simulink model "closed_loop_pd"  (R2023b)
settings: Solver=VariableStepAuto  StartTime=0.0  StopTime=0.15  RelTol=1e-3
undefined symbols (not defined in the file): a_m, config, K, K_g, K_m, K_pot, Kpd
settings Model: Creator=foderking  LastModifiedBy=foderking

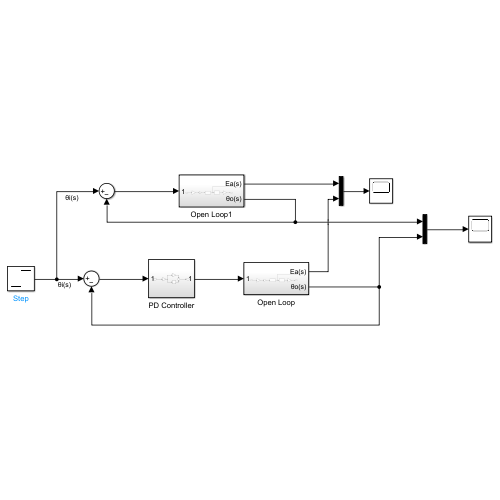
[thumbnail: Simulink's stored preview of the top-level diagram]
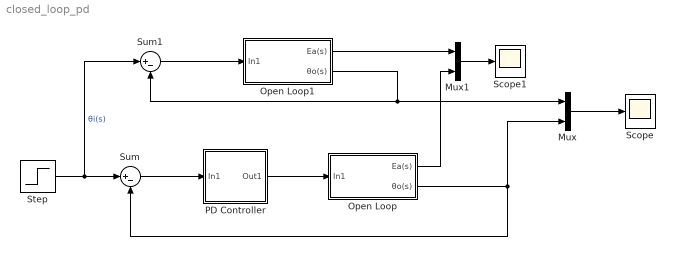
== system closed_loop_pd ==
  Mux : Mux  Inputs=2
  Mux1 : Mux  Inputs=2
  Open Loop : Subsystem
  Open Loop1 : Subsystem
  PD Controller : Subsystem
  Scope : Scope
  Scope1 : Scope
  Step : Step  Time=0  SampleTime=0
  Sum : Sum  Inputs=|+-
  Sum1 : Sum  Inputs=|+-
  wires:
  Open Loop/2(θo(s)) -> Sum/2, Mux/2
  Open Loop/1(Ea(s)) -> Mux1/2
  Step/1 -> Sum1/1, Sum/1  "θi(s)"
  Sum1/1 -> Open Loop1/1(In1)
  Open Loop1/1(Ea(s)) -> Mux1/1
  Open Loop1/2(θo(s)) -> Mux/1, Sum1/2
  Mux/1 -> Scope/1
  Sum/1 -> PD Controller/1(In1)
  PD Controller/1(Out1) -> Open Loop/1(In1)
  Mux1/1 -> Scope1/1

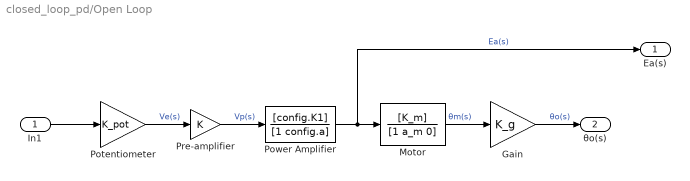
== system closed_loop_pd/Open Loop ==
  In1 : Inport
  Gain : Gain  Gain=K_g
  Motor : TransferFcn  Numerator=[K_m]  Denominator=[1 a_m 0]
  Potentiometer : Gain  Gain=K_pot
  Power Amplifier : TransferFcn  Numerator=[config.K1]  Denominator=[1 config.a]
  Pre-amplifier : Gain  Gain=K
  Ea(s) : Outport
  θo(s) : Outport  Port=2
  wires:
  Power Amplifier/1 -> Ea(s)/1, Motor/1  "Ea(s)"
  Potentiometer/1 -> Pre-amplifier/1  "Ve(s)"
  Motor/1 -> Gain/1  "θm(s)"
  In1/1 -> Potentiometer/1
  Pre-amplifier/1 -> Power Amplifier/1  "Vp(s)"
  Gain/1 -> θo(s)/1  "θo(s)"

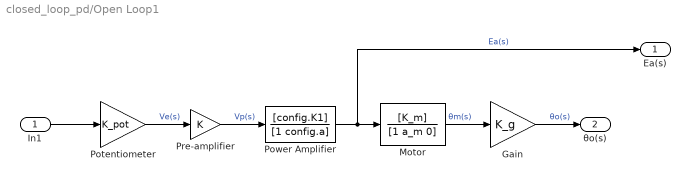
== system closed_loop_pd/Open Loop1 ==
  In1 : Inport
  Gain : Gain  Gain=K_g
  Motor : TransferFcn  Numerator=[K_m]  Denominator=[1 a_m 0]
  Potentiometer : Gain  Gain=K_pot
  Power Amplifier : TransferFcn  Numerator=[config.K1]  Denominator=[1 config.a]
  Pre-amplifier : Gain  Gain=K
  Ea(s) : Outport
  θo(s) : Outport  Port=2
  wires:
  Power Amplifier/1 -> Ea(s)/1, Motor/1  "Ea(s)"
  Potentiometer/1 -> Pre-amplifier/1  "Ve(s)"
  Motor/1 -> Gain/1  "θm(s)"
  In1/1 -> Potentiometer/1
  Pre-amplifier/1 -> Power Amplifier/1  "Vp(s)"
  Gain/1 -> θo(s)/1  "θo(s)"

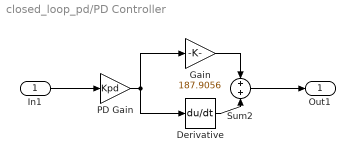
== system closed_loop_pd/PD Controller ==
  In1 : Inport
  Derivative : Derivative
  Gain : Gain  Gain=187.9056
  PD Gain : Gain  Gain=Kpd
  Sum2 : Sum  Inputs=+|+
  Out1 : Outport
  wires:
  Gain/1 -> Sum2/1
  In1/1 -> PD Gain/1
  Derivative/1 -> Sum2/2
  PD Gain/1 -> Derivative/1, Gain/1
  Sum2/1 -> Out1/1
